simulink model "moxingxitong2zenjiafadianjizhuandongguanliang"  (Simulink 7.4)
settings: Solver=ode15s  StartTime=0.0  StopTime=30  RelTol=1e-3
undefined symbols (not defined in the file or in its folder): D1, Delta
libraries: powerlib x17
settings Model: Creator=admini  LastModifiedBy=admini
settings DataIOCC: SaveFinalState=on

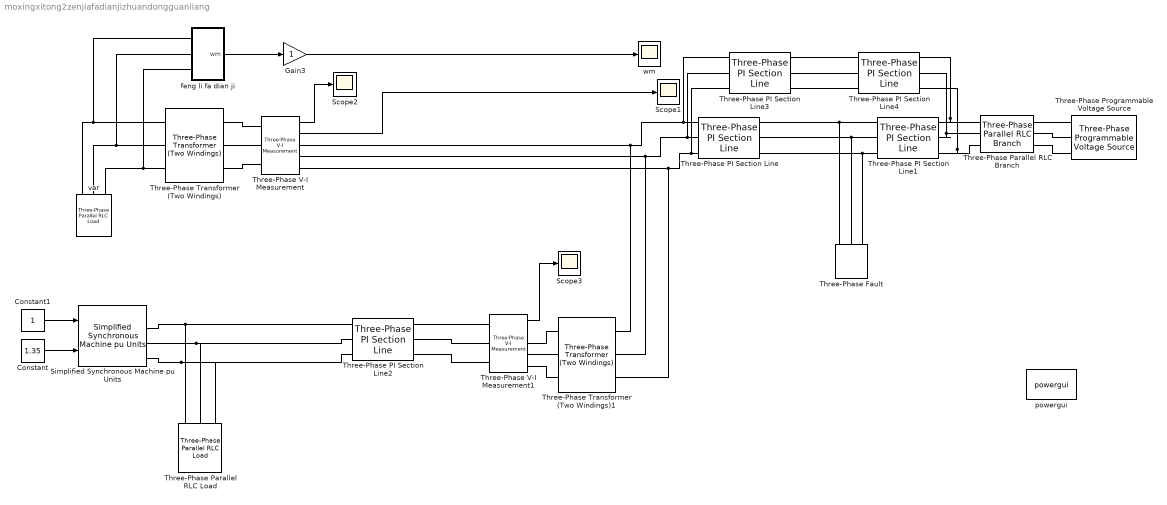
== system moxingxitong2zenjiafadianjizhuandongguanliang ==
  Constant : Constant  Value=1.35  OutDataType=fixdt(1, 16)  OutScaling=2^0
  Constant1 : Constant  OutDataType=fixdt(1, 16)  OutScaling=2^0
  Gain3 : Gain  ParameterDataType=fixdt(1, 16)  ParameterScaling=2^0  OutDataType=fixdt(1, 16)  OutScaling=2^0
  Scope1 : Scope
      settings: TimeRange=0.1  YMin=-800  YMax=800
  Scope2 : Scope
      settings: TimeRange=0.1  YMin=-50000  YMax=50000  SaveName=ScopeData2
  Scope3 : Scope
      settings: TimeRange=10  YMin=-10000  YMax=12000  SaveName=ScopeData7
  Simplified Synchronous Machine pu Units : powerlib/Machines/Simplified Synchronous Machine pu Units  DialogController=POWERSYS.PowerSysDialog  SystemSampleTime=-1  ConnectionType=3-wire Y  MechanicalLoad=Mechanical power Pm  NominalParameters=[200e6 13800 50]  Mechanical=[3.7 0 20]  InternalRL="[0.02  0.3]"  InitialConditions="[ 0,0   0,0,0   0,0,0 ]"  Units=0  LoadFlowParameters=[1,0,0,0,0]  TsPowergui=0  TsBlock=-1
  Three-Phase PI Section Line{,1..4} (5 alike) : powerlib/Elements/Three-Phase PI Section Line  DialogController=POWERSYS.PowerSysDialog  PhysicalDomain=powersysdomain  SubClassName=unknown  LeftPortType=p1  RightPortType=p1  LConnTagsString=a|b|c  RConnTagsString=A|B|C  Frequency=50  Resistances=[ 0.01273 0.3864]  Inductances="[ 0.9337e-3  4.1264e-3]"  Capacitances=[12.74e-9 7.751e-9]  Length=100
  Three-Phase Parallel RLC Branch : powerlib/Elements/Three-Phase Parallel RLC Branch  DialogController=POWERSYS.PowerSysDialog  PhysicalDomain=powersysdomain  SubClassName=unknown  LeftPortType=p1  RightPortType=p1  LConnTagsString=A|B|C  RConnTagsString=A|B|C  BranchType=R  Resistance=1.0  Inductance=1.0  Capacitance=1.0  Measurements=None
  Three-Phase Parallel RLC Load : powerlib/Elements/Three-Phase Parallel RLC Load  DialogController=POWERSYS.PowerSysDialog  PhysicalDomain=powersysdomain  SubClassName=unknown  LeftPortType=p1  RightPortType=p1  LConnTagsString=A|B|C  Configuration=Y (grounded)  NominalVoltage=1000  NominalFrequency=60  ActivePower=500e3  InductivePower=100  CapacitivePower=0  Measurements=None
  Three-Phase Programmable Voltage Source : powerlib/Electrical Sources/Three-Phase Programmable Voltage Source  DialogController=POWERSYS.PowerSysDialog  SystemSampleTime=-1  PositiveSequence="[66000  0 50]"  VariationEntity=None  VariationType=Step  VariationStep=0.5  VariationRate=10  VariationMagnitude=0.3  VariationFrequency=2  VariationTiming=[1 2]  VariationPhaseA=off  Amplitudes=[1 0.8 1.2 1.0]  TimeValues=[0 0.1 0.15 0.2]  HarmonicGeneration=off  HarmonicA=[3 0.2 -25 0]  HarmonicB=[2 0.15 35 2]  Timing="[0.05  3]"
  Three-Phase Transformer (Two Windings) : powerlib/Elements/Three-Phase Transformer (Two Windings)  DialogController=POWERSYS.PowerSysDialog  SystemSampleTime=-1  Winding1Connection=Delta (D1)  UNITS=pu  NominalPower=[ 250e6 , 50 ]  Winding1=[ 400 , 0.002 , 0.08 ]  Winding2Connection=Yg  Winding2=[ 66000 , 0.002 , 0.08 ]  SetSaturation=off  Rm=500  Lm=500  Saturation=[ 0,0 ; 0.0024,1.2 ; 1.0,1.52 ]  Hysteresis=off  DataFile='hysteresis'  SetInitialFlux=off  InitialFluxes=[ 0.8 , -0.8 , 0.7 ]  Measurements=None  MoreParameters=off  BreakLoop=off  DataType=off  TransfoNumber=1
  Three-Phase Transformer (Two Windings)1 : powerlib/Elements/Three-Phase Transformer (Two Windings)  DialogController=POWERSYS.PowerSysDialog  SystemSampleTime=-1  Winding1Connection=Delta (D1)  UNITS=pu  NominalPower=[ 250e6 , 50 ]  Winding1=[ 13800 , 0.002 , 0.08 ]  Winding2Connection=Yg  Winding2=[ 66000 , 0.002 , 0.08 ]  SetSaturation=off  Rm=500  Lm=500  Saturation=[ 0,0 ; 0.0024,1.2 ; 1.0,1.52 ]  Hysteresis=off  DataFile='hysteresis'  SetInitialFlux=off  InitialFluxes=[ 0.8 , -0.8 , 0.7 ]  Measurements=None  MoreParameters=off  BreakLoop=off  DataType=off  TransfoNumber=1
  Three-Phase V-I Measurement : powerlib/Measurements/Three-Phase V-I Measurement  DialogController=POWERSYS.PowerSysDialog  SystemSampleTime=-1  VoltageMeasurement=phase-to-ground  SetLabelV=off  LabelV=Vabc  Vpu=off  CurrentMeasurement=yes  SetLabelI=off  LabelI=Iabc  Ipu=off  Pbase=100e6  Vbase=500e3  OutputType=Complex  PhasorSimulation=off  PSBequivalent=0
  Three-Phase V-I Measurement1 : powerlib/Measurements/Three-Phase V-I Measurement  DialogController=POWERSYS.PowerSysDialog  SystemSampleTime=-1  VoltageMeasurement=phase-to-ground  SetLabelV=off  LabelV=Vabc  Vpu=off  CurrentMeasurement=yes  SetLabelI=off  LabelI=Iabc  Ipu=off  Pbase=100e6  Vbase=500e3  OutputType=Complex  PhasorSimulation=off  PSBequivalent=0
  Three-Phase Fault : powerlib/Elements/Three-Phase Fault  DialogController=POWERSYS.PowerSysDialog  SystemSampleTime=-1  FaultA=on  FaultB=on  FaultC=on  FaultResistance=0.001  GroundFault=on  GroundResistance=0.001  External=off  SwitchStatus=[1 0]  SwitchTimes=[10 10.2]  InitialStates=[0 0 1]  SnubberResistance=1e6  SnubberCapacitance=inf  Measurements=None
  feng li fa dian ji : Subsystem
  powergui : powerlib/powergui  Priority=1  SystemSampleTime=-1  SimulationMode=Continuous  SampleTime=50e-6  frequency=50  SPID=off  DisableSnubberDevices=off  DisableRonSwitches=off  DisableVfSwitches=off  SwTol=0  Interpol=off  frequencyindice=50  echomessages=off  HookPort=off  DisplayEquations=off  FunctionMessages=off  EnableUseOfTLC=off  x0status=blocks  RestoreLinks=warning  Frange=[0:2:500]  Ylog=off  Xlog=on  ShowGrid=off  save=off  variable=ZData  ZoomFFT=on  StartTime=0.0  cycles=1  DisplayStyle=1  fundamental=60  FreqAxis=off  MaxFrequency=1000  frequencyindicesteady=1  RmsSteady=1  display=off  Ts=0  methode=off
  var : powerlib/Elements/Three-Phase Parallel RLC Load  DialogController=POWERSYS.PowerSysDialog  PhysicalDomain=powersysdomain  SubClassName=unknown  LeftPortType=p1  RightPortType=p1  LConnTagsString=A|B|C  Configuration=Delta  NominalVoltage=400  NominalFrequency=50  ActivePower=0  InductivePower=0  CapacitivePower=10000e3  Measurements=None
  wm : Scope
      settings: TimeRange=10  YMin=-0.03  YMax=0.035  SaveName=lpy  DataFormat=Array
  wires:
  Three-Phase V-I Measurement/1 -> Scope2/1
  Three-Phase V-I Measurement/2 -> Scope1/1
  feng li fa dian ji/1(wm) -> Gain3/1
  Gain3/1 -> wm/1
  Three-Phase V-I Measurement1/1 -> Scope3/1
  Constant1/1 -> Simplified Synchronous Machine pu Units/1
  Constant/1 -> Simplified Synchronous Machine pu Units/2
  connections:
  Three-Phase Transformer (Two Windings)/LConn1 -- var/LConn1 -- feng li fa dian ji/LConn1
  var/LConn2 -- Three-Phase Transformer (Two Windings)/LConn2 -- feng li fa dian ji/LConn2
  Three-Phase Transformer (Two Windings)/LConn3 -- var/LConn3 -- feng li fa dian ji/LConn3
  Three-Phase Transformer (Two Windings)1/RConn1 -- Three-Phase V-I Measurement/RConn1 -- Three-Phase PI Section Line/LConn1 -- Three-Phase PI Section Line3/LConn1
  Three-Phase Transformer (Two Windings)1/RConn2 -- Three-Phase V-I Measurement/RConn2 -- Three-Phase PI Section Line/LConn2 -- Three-Phase PI Section Line3/LConn2
  Three-Phase Transformer (Two Windings)1/RConn3 -- Three-Phase V-I Measurement/RConn3 -- Three-Phase PI Section Line/LConn3 -- Three-Phase PI Section Line3/LConn3
  Three-Phase PI Section Line4/RConn1 -- Three-Phase Parallel RLC Branch/LConn1 -- Three-Phase PI Section Line1/RConn1
  Three-Phase PI Section Line4/RConn2 -- Three-Phase Parallel RLC Branch/LConn2 -- Three-Phase PI Section Line1/RConn2
  Three-Phase PI Section Line1/RConn3 -- Three-Phase PI Section Line4/RConn3 -- Three-Phase Parallel RLC Branch/LConn3
  Three-Phase PI Section Line1/LConn2 -- Three-Phase PI Section Line/RConn2 -- Three-Phase Fault/LConn2
  Three-Phase Fault/LConn1 -- Three-Phase PI Section Line/RConn1 -- Three-Phase PI Section Line1/LConn1
  Three-Phase PI Section Line1/LConn3 -- Three-Phase PI Section Line/RConn3 -- Three-Phase Fault/LConn3
  Three-Phase Parallel RLC Load/LConn3 -- Three-Phase PI Section Line2/LConn3 -- Simplified Synchronous Machine pu Units/RConn3
  Three-Phase Parallel RLC Load/LConn2 -- Three-Phase PI Section Line2/LConn2 -- Simplified Synchronous Machine pu Units/RConn2
  Three-Phase Parallel RLC Load/LConn1 -- Three-Phase PI Section Line2/LConn1 -- Simplified Synchronous Machine pu Units/RConn1
  Three-Phase Transformer (Two Windings)/RConn1 -- Three-Phase V-I Measurement/LConn1
  Three-Phase Transformer (Two Windings)/RConn2 -- Three-Phase V-I Measurement/LConn2
  Three-Phase Transformer (Two Windings)/RConn3 -- Three-Phase V-I Measurement/LConn3
  Three-Phase PI Section Line3/RConn1 -- Three-Phase PI Section Line4/LConn1
  Three-Phase PI Section Line3/RConn2 -- Three-Phase PI Section Line4/LConn2
  Three-Phase PI Section Line3/RConn3 -- Three-Phase PI Section Line4/LConn3
  Three-Phase V-I Measurement1/RConn1 -- Three-Phase Transformer (Two Windings)1/LConn1
  Three-Phase V-I Measurement1/RConn2 -- Three-Phase Transformer (Two Windings)1/LConn2
  Three-Phase V-I Measurement1/RConn3 -- Three-Phase Transformer (Two Windings)1/LConn3
  Three-Phase PI Section Line2/RConn1 -- Three-Phase V-I Measurement1/LConn1
  Three-Phase PI Section Line2/RConn2 -- Three-Phase V-I Measurement1/LConn2
  Three-Phase PI Section Line2/RConn3 -- Three-Phase V-I Measurement1/LConn3
  Three-Phase Parallel RLC Branch/RConn1 -- Three-Phase Programmable Voltage Source/RConn1
  Three-Phase Parallel RLC Branch/RConn2 -- Three-Phase Programmable Voltage Source/RConn2
  Three-Phase Parallel RLC Branch/RConn3 -- Three-Phase Programmable Voltage Source/RConn3

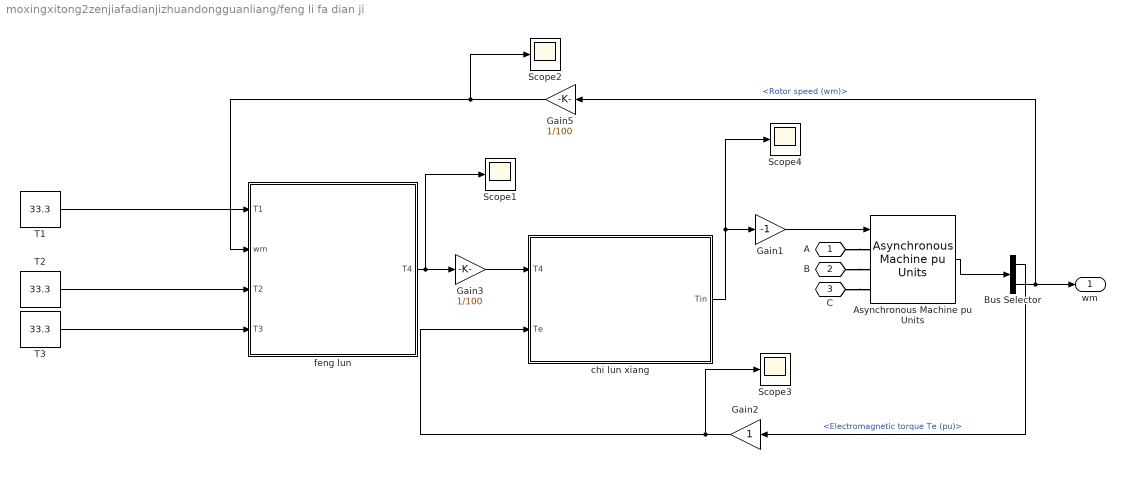
== system moxingxitong2zenjiafadianjizhuandongguanliang/feng li fa dian ji ==
  Asynchronous Machine pu Units : powerlib/Machines/Asynchronous Machine pu Units  DialogController=POWERSYS.PowerSysDialog  SystemSampleTime=-1  PresetModel=No  MechanicalLoad=Torque Tm  ShowDetailedParameters=on  RotorType=Squirrel-cage  ReferenceFrame=Rotor  NominalParameters=[50000000 400 50]  Stator=[0.01379 0.04775]  Rotor=[0.007728 0.04775]  Lm=2.416  Mechanical=[0.1419 0.008726 2]  PolePairs=2  InitialConditions="[ 1,0   1,1,1  0,0,0 ]"  Units=pu  LoadFlowParameters=0  SimulateSaturation=off  Saturation="[0.212,0.4201,0.8125,1.0979,1.4799,2.2457,3.2586,4.5763,6.4763 ;   0.5,0.7,0.9,1,1.1,1.2 ,1.3,1.4,1.5]"  TsPowergui=0  TsBlock=-1  IterativeModel=Forward Euler
      link override Electrical model/Continuous/Stator/phiqs: InitialCondition=0.00001
      link override Mechanical model/Continuous Tm input/Rotor angle thetam: InitialCondition=0.0001
      link override Mechanical model/Continuous Tm input/Rotor speed (wm): InitialCondition=0.0001
  Bus Selector : BusSelector  OutputSignals=Mechanical.Electromagnetic torque Te (pu),Mechanical.Rotor speed (wm)
  Gain1 : Gain  Gain=-1  ParameterDataType=fixdt(1, 16)  ParameterScaling=2^0  OutDataType=fixdt(1, 16)  OutScaling=2^0
  Gain2 : Gain  ParameterDataType=fixdt(1, 16)  ParameterScaling=2^0  OutDataType=fixdt(1, 16)  OutScaling=2^0
  Gain3 : Gain  Gain=1/100  ParameterDataType=fixdt(1, 16)  ParameterScaling=2^0  OutDataType=fixdt(1, 16)  OutScaling=2^0
  Gain5 : Gain  Gain=1/100  ParameterDataType=fixdt(1, 16)  ParameterScaling=2^0  OutDataType=fixdt(1, 16)  OutScaling=2^0
  Scope{1..4} (4 alike) : Scope
      Scope1 settings: TimeRange=10  YMin=-4500  YMax=5000  SaveName=ScopeData4
      Scope2 settings: TimeRange=0.1  YMin=-0.0004  YMax=7.5e-005  SaveName=ScopeData3
      Scope3 settings: TimeRange=0.1  YMin=-3.75  YMax=0.5  SaveName=ScopeData5
      Scope4 settings: TimeRange=0.1  YMin=-0.15  YMax=0.4  SaveName=ScopeData6
  T1 : Constant  Value=33.3  OutDataType=fixdt(1, 16)  OutScaling=2^0
  T2 : Constant  Value=33.3  OutDataType=fixdt(1, 16)  OutScaling=2^0
  T3 : Constant  Value=33.3  OutDataType=fixdt(1, 16)  OutScaling=2^0
  chi lun xiang : Subsystem
  feng lun : Subsystem
  A : PMIOPort  Port=1  Side=Left
  B : PMIOPort  Port=2  Side=Left
  C : PMIOPort  Port=3  Side=Left
  wm : Outport
  wires:
  Asynchronous Machine pu Units/1 -> Bus Selector/1
  Bus Selector/2 -> wm/1, Gain5/1  "<Rotor speed (wm)>"
  T2/1 -> feng lun/3(T2)
  T3/1 -> feng lun/4(T3)
  T1/1 -> feng lun/1(T1)
  chi lun xiang/1(Tin) -> Gain1/1, Scope4/1
  Bus Selector/1 -> Gain2/1  "<Electromagnetic torque Te (pu)>"
  Gain2/1 -> chi lun xiang/2(Te), Scope3/1
  Gain5/1 -> feng lun/2(wm), Scope2/1
  feng lun/1(T4) -> Gain3/1, Scope1/1
  Gain3/1 -> chi lun xiang/1(T4)
  Gain1/1 -> Asynchronous Machine pu Units/1
  connections:
  A/RConn1 -- Asynchronous Machine pu Units/LConn1
  B/RConn1 -- Asynchronous Machine pu Units/LConn2
  C/RConn1 -- Asynchronous Machine pu Units/LConn3

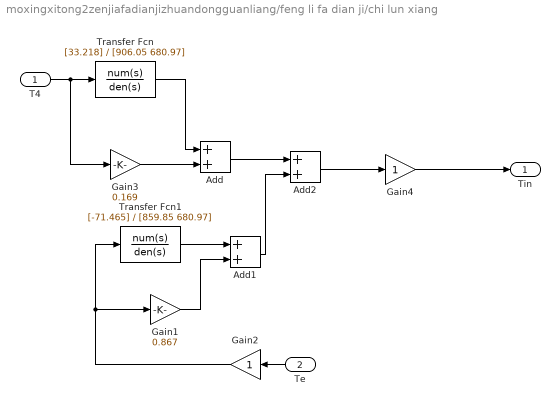
== system moxingxitong2zenjiafadianjizhuandongguanliang/feng li fa dian ji/chi lun xiang ==
  T4 : Inport
  Te : Inport  Port=2
  Add : Sum  OutDataType=fixdt(1, 16)  OutScaling=2^-10
  Add1 : Sum  OutDataType=fixdt(1, 16)  OutScaling=2^-10
  Add2 : Sum  OutDataType=fixdt(1, 16)  OutScaling=2^-10
  Gain1 : Gain  Gain=0.867  ParameterDataType=fixdt(1, 16)  ParameterScaling=2^0  OutDataType=fixdt(1, 16)  OutScaling=2^0
  Gain2 : Gain  ParameterDataType=fixdt(1, 16)  ParameterScaling=2^0  OutDataType=fixdt(1, 16)  OutScaling=2^0
  Gain3 : Gain  Gain=0.169  ParameterDataType=fixdt(1, 16)  ParameterScaling=2^0  OutDataType=fixdt(1, 16)  OutScaling=2^0
  Gain4 : Gain  ParameterDataType=fixdt(1, 16)  ParameterScaling=2^0  OutDataType=fixdt(1, 16)  OutScaling=2^0
  Transfer Fcn : TransferFcn  Numerator=[33.218]  Denominator=[906.05 680.97]  AbsoluteTolerance=0.01
  Transfer Fcn1 : TransferFcn  Numerator=[-71.465]  Denominator=[859.85 680.97]  AbsoluteTolerance=0.01
  Tin : Outport
  wires:
  Transfer Fcn/1 -> Add/1
  Transfer Fcn1/1 -> Add1/1
  Add/1 -> Add2/1
  Add1/1 -> Add2/2
  Gain3/1 -> Add/2
  Gain1/1 -> Add1/2
  Gain2/1 -> Transfer Fcn1/1, Gain1/1
  Add2/1 -> Gain4/1
  Gain4/1 -> Tin/1
  T4/1 -> Gain3/1, Transfer Fcn/1
  Te/1 -> Gain2/1

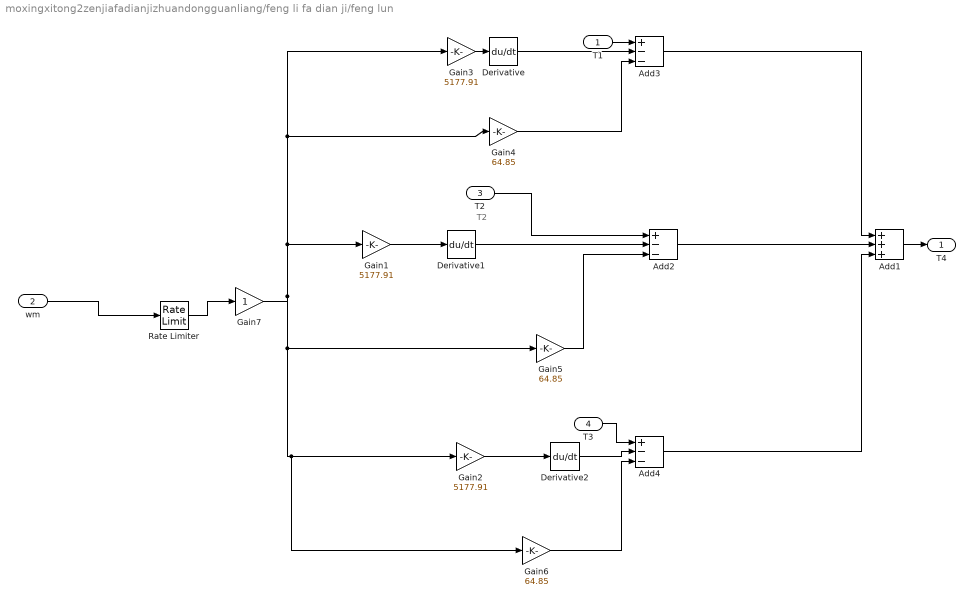
== system moxingxitong2zenjiafadianjizhuandongguanliang/feng li fa dian ji/feng lun ==
  note: T2
  T1 : Inport
  wm : Inport  Port=2  OutDataType=fixdt(1, 16)  OutScaling=2^0
  T2 : Inport  Port=3
  T3 : Inport  Port=4
  Add1 : Sum  Inputs=+++  OutDataType=fixdt(1, 16)  OutScaling=2^-10
  Add2 : Sum  Inputs=+--  OutDataType=fixdt(1, 16)  OutScaling=2^-10
  Add3 : Sum  Inputs=+--  OutDataType=fixdt(1, 16)  OutScaling=2^-10
  Add4 : Sum  Inputs=+--  OutDataType=fixdt(1, 16)  OutScaling=2^-10
  Derivative : Derivative
  Derivative1 : Derivative
  Derivative2 : Derivative
  Gain1 : Gain  Gain=5177.91  ParameterDataType=fixdt(1, 16)  ParameterScaling=2^0  OutDataType=fixdt(1, 16)  OutScaling=2^0
  Gain2 : Gain  Gain=5177.91  ParameterDataType=fixdt(1, 16)  ParameterScaling=2^0  OutDataType=fixdt(1, 16)  OutScaling=2^0
  Gain3 : Gain  Gain=5177.91  ParameterDataType=fixdt(1, 16)  ParameterScaling=2^0  OutDataType=fixdt(1, 16)  OutScaling=2^0
  Gain4 : Gain  Gain=64.85  ParameterDataType=fixdt(1, 16)  ParameterScaling=2^0  OutDataType=fixdt(1, 16)  OutScaling=2^0
  Gain5 : Gain  Gain=64.85  ParameterDataType=fixdt(1, 16)  ParameterScaling=2^0  OutDataType=fixdt(1, 16)  OutScaling=2^0
  Gain6 : Gain  Gain=64.85  ParameterDataType=fixdt(1, 16)  ParameterScaling=2^0  OutDataType=fixdt(1, 16)  OutScaling=2^0
  Gain7 : Gain  ParameterDataType=fixdt(1, 16)  ParameterScaling=2^0  OutDataType=fixdt(1, 16)  OutScaling=2^0
  Rate Limiter : RateLimiter  RisingSlewLimit=100  FallingSlewLimit=-100  SampleTimeMode=inherited  LinearizeAsGain=off
  T4 : Outport
  wires:
  Add3/1 -> Add1/1
  Add4/1 -> Add1/3
  Gain3/1 -> Derivative/1
  Derivative/1 -> Add3/2
  Gain1/1 -> Derivative1/1
  Gain2/1 -> Derivative2/1
  Derivative2/1 -> Add4/2
  Add2/1 -> Add1/2
  Gain4/1 -> Add3/3
  Gain6/1 -> Add4/3
  Add1/1 -> T4/1
  Gain7/1 -> Gain1/1, Gain3/1, Gain4/1, Gain2/1, Gain6/1, Gain5/1
  T1/1 -> Add3/1
  T3/1 -> Add4/1
  T2/1 -> Add2/1
  Derivative1/1 -> Add2/2
  Gain5/1 -> Add2/3
  wm/1 -> Rate Limiter/1
  Rate Limiter/1 -> Gain7/1
